simulink model "ClosedLoopControl"  (R2016b)
settings: Solver=FixedStepDiscrete  StartTime=0.0  StopTime=Inf  FixedStep=sCoreParams.core.stepPeriod  RelTol=1e-3  EnableMultiTasking=on
undefined symbols (not defined in the file): fdesignblkfcn, gcbh, High, sCoreParams, sCoreParams_decoders_chanceDetector_randStimEventsPerSec, sCoreParams_decoders_txDetector_channel1, sCoreParams_decoders_txDetector_channel2, sCoreParams_decoders_txDetector_detectChannelInds, sCoreParams_decoders_txDetector_nChannels, sCoreParams_Features_Baseline_initialThresholdValue, sCoreParams_Features_Baseline_weightPreviousThreshold, sCoreParams_Features_Data_SmoothWindowsDurationSamples, sCoreParams_stimulator_stimAfterDelaySteps
libraries: dsparch4 x20, dspstat3 x19, dspspect3 x6, dspfdesign x2, dspindex x2, dspswit3 x1
(part 3 of 6)

== system ClosedLoopControl/FilterBanks/Variant FILTER 1000/4-8Hz Theta FIR ==
  EEGData : Inport
  Generated Filter Block : DiscreteFir  Tag=BlockMethodSubSystem  Coefficients=[-4.0965914206968854e-05 -3.1562576663732106e-05 -2.1885911724999518e-05 -1.1939596349254351e-05 -1.7275529186717732e-06 8.7460521918561927e-06 1.947681025149899e-05 3.0460072015961004e-05 4.1690949775364282e-05 5.316431960704088e-05 6.4874823832640496e-05 7.6816873678724166e-05 8.8984652139878232e-05 0.00010137211704322235 0.00011397300431296607 0.00012678083143356132 0.00013978890110980167 0.00015299030512201677 0.0001663779283744122 0.00017994445313437968 0.00019368236346045136 0.00020758394981644162 0.00022164131386907284 0.00023584637346632409 0.00025019086779349122 0.00026466636270383186 0.00027926425622051192 0.00029397578420637229 0.0003087920261979428 0.00032370391139992542 0.00033870222483622773 0.00035377761365352274 0.00036892059357309124 0.00038412155548662883 0.00039937077219152613 0.00041465840526098188 0.00042997451204421873 0.00044530905279189289 0.00046065189790167919 0.00047599283527891651 0.00049132157780700891 0.00050662777092225068 0.00052190100028754523 0.00053713079955942423 0.0005523066582426813 0.00056741802962677009 0.00058245433879808891 0.000597404990722145 0.00061225937838948802 0.00062700689101926807 0.00064163692231413751 0.0006561388787601712 0.00067050218796541777 0.00068471630703058827 0.00069877073094537284 0.00071265500100379619 0.00072635871323196185 0.00073987152682152089 0.00075318317256212598 0.00076628346126611058 0.00077916229217862127 0.00079180966136635381 0.00080421567007808498 0.00081637053307013834 0.00082826458688991199 0.00083988829811062636 0.0008512322715104072 0.00086228725818885592 0.00087304416361427394 0.00088349405559469028 0.00089362817216592349 0.00090343792938986952 0.00091291492905630825 0.00092205096628152127 0.00093083803699705442 0.0009392683453220477 0.00094733431081258041 0.00095502857558154447 0.00096234401128264535 0.00096927372595218225 0.00097581107070235091 0.0009819496462598993 0.00098768330934403915 0.00099300617887762544 0.00099791264202572761 0.0010023973600557757 0.0010064552740136482 0.0010100816102101011 0.0010132718855121318 0.001016021912433947 0.0010183278040223579 0.0010201859785315629 0.001021593163882393 0.0010225464019012794 0.0010230430523343159 0.0010230807966319598 0.0010226576415000763 0.0010217719222131735 0.0010204223056858744 0.0010186077932988016 0.0010163277234752684 0.0010135817740053027 0.001010369964113756 0.0010066926562693997 0.0010025505577321177 0.00099794472183549455 0.00099287654900228565 0.00098734778749046018 0.00098136053386771059 0.00097491723321251631 0.00096802067904005952 0.00096067401295151704 0.00095288072400541532 0.0009446446478100181 0.0009359699653358561 0.00092686120144778344 0.0009173232231561401 0.00090736123758679863 0.00089698078967015025 0.00088618775954923501 0.00087498835970750667 0.00086338913181691805 0.00085139694330722165 0.00083901898365764142 0.00082626276041227885 0.00081313609492081231 0.00079964711780634835 0.00078580426416241132 0.00077161626848136554 0.0007570921593167498 0.00074224125368220961 0.00072707315118998063 0.00071159772793206099 0.00069582513010743195 0.00067976576739893664 0.00066343030610358899 0.00064682966202034113 0.00062997499309955815 0.0006128776918585834 0.00059554937756810765 0.00057800188821412754 0.00056024727224058429 0.00054229778007792984 0.00052416585546304225 0.00050586412655614986 0.00048740539686060552 0.00046880263595147945 0.00045006897001921846 0.00043121767223470618 0.00041226215294230351 0.00039321594968756213 0.00037409271708650435 0.00035490621654351472 0.0003356703058250473 0.00031639892849649162 0.00029710610322969557 0.00027780591298878944 0.00025851249410209314 0.0002392400252279985 0.00022000271622286136 0.00020081479691906072 0.00018169050582149475 0.00016264407873087066 0.00014368973730227231 0.00012484167754757907 0.00010611405829039998 8.7520989582255267e-05 6.9076521088845522e-05 5.0794630455274516e-05 3.268921165922444e-05 1.4774063361054236e-05 -2.937122740077089e-06 -2.0430773534982893e-05 -3.7693446108933282e-05 -5.4711839312708335e-05 ...(+22999 chars)]  InputProcessing=Columns as channels (frame based)
  filteredData : Outport
  wires:
  EEGData/1 -> Generated Filter Block/1
  Generated Filter Block/1 -> filteredData/1

== system ClosedLoopControl/FilterBanks/Variant FILTER 1000/4-8Hz Theta IIR ==
  EEGData : Inport
  Generated Filter Block : dsparch4/Biquad Filter  Tag=BlockMethodSubSystem  IIRFiltStruct=Direct form II  CoeffSource=Specify via dialog  BiQuadCoeffs=[0.06931048107077438 0 -0.06931048107077438 1 -1.9802222626264796 0.98069219275950414;0.018212718480246574 0 -0.018212718480246574 1 -1.974229549932226 0.97738422717098938;0.023158348233385473 0 -0.023158348233385473 1 -1.9641498959199661 0.96500779271339332;0.0024959904089144444 0 -0.0024959904089144444 1 -1.9561756271771134 0.95744921192041055;0.0038077695663208747 0 -0.0038077695663208747 1 -1.997161027977103 0.9974982403948508;0.014974735737014893 0 -0.014974735737014893 1 -1.9920313655652335 0.99238598997351135;0.067760808502200814 0 -0.067760808502200814 1 -1.9727869770434667 0.9733937566537022;0.057203187978703156 0 -0.057203187978703156 1 -1.9624464044097747 0.96525472973103199;0.04408340167774278 0 -0.04408340167774278 1 -1.9548134348661885 0.95715627089409527;0.057491867954990714 0 -0.057491867954990714 1 -1.9525307286276412 0.95433606793971626;0.0088260244022239226 0 -0.0088260244022239226 1 -1.9887766913282909 0.99212744222685822;2 0 -2 1 -1.9865011906165977 0.98689604525630514]  a0Flag=Warning  IC=0  ICnum=0  ICden=0  InputProcessing=Columns as channels (frame based)  denAccumFracLength=30  denProdOutputFracLength=30  secondMemoryFracLength=15  roundingMode=Floor  overflowMode=off  ScaleValues=[0.00037611451030394085;1;1;1;1;1;1;1;1;1;1;1;12.523892689936686]  optimizeScaleValues=off  ScaleValueMode=Specify via input port (g)  scaleValueFracLength=14  FilterSource=Specify via dialog  FilterObject=BQF
  filteredData : Outport
  wires:
  EEGData/1 -> Generated Filter Block/1
  Generated Filter Block/1 -> filteredData/1

== system ClosedLoopControl/FilterBanks/Variant FILTER 1000/65-110Hz HighGamma FIR ==
  EEGData : Inport
  Generated Filter Block : DiscreteFir  Tag=BlockMethodSubSystem  Coefficients=[0.013804330140111717 -0.0032030301327593746 -0.0026076510316669732 -0.0019065599324483403 -0.0010950973516722739 -0.00016216284695244599 0.00086566972400229725 0.0019516885555648496 0.0030106913379105565 0.0039390669121143725 0.0046071460998753817 0.0048943907316536354 0.0046884459511977224 0.0039269229728160996 0.0025931297718577782 0.00075000967683423552 -0.0014812603255484518 -0.0039070830585515659 -0.0062985241582419948 -0.0083973498946592028 -0.0099678263784681084 -0.010809035903715401 -0.010803230740337099 -0.0099149025044472407 -0.0082222253166924462 -0.0058958474615859622 -0.0031966951596653086 -0.00042921572872034144 0.0020843075499259859 0.0040591524840028152 0.005272016533938776 0.0056235264011517839 0.0051356663591639361 0.0039469466526657771 0.0023736337698522614 0.00069406556447416045 -0.00062224964462739992 -0.0012265818590162169 -0.00086373706682174275 0.00064926343879799649 0.0032891772017854025 0.0068616007904351807 0.010959888764209976 0.015047965951643011 0.018483860601451012 0.020629088707457537 0.020895258620364673 0.018864941232038121 0.014327792052099074 0.0073683568396857536 -0.0016488647216768106 -0.012058123582057797 -0.022974047895930626 -0.033340495226029006 -0.042069205650392676 -0.048123624580120594 -0.050670829782113042 -0.04915218268598933 -0.043397073906481516 -0.033631108507841165 -0.020501148353700021 -0.0049965672361083416 0.011603807282296149 0.02788293342498982 0.042383528564973294 0.053814263792701968 0.061127840120098795 0.06363510173931633 0.061127840120098795 0.053814263792701968 0.042383528564973294 0.02788293342498982 0.011603807282296149 -0.0049965672361083416 -0.020501148353700021 -0.033631108507841165 -0.043397073906481516 -0.04915218268598933 -0.050670829782113042 -0.048123624580120594 -0.042069205650392676 -0.033340495226029006 -0.022974047895930626 -0.012058123582057797 -0.0016488647216768106 0.0073683568396857536 0.014327792052099074 0.018864941232038121 0.020895258620364673 0.020629088707457537 0.018483860601451012 0.015047965951643011 0.010959888764209976 0.0068616007904351807 0.0032891772017854025 0.00064926343879799649 -0.00086373706682174275 -0.0012265818590162169 -0.00062224964462739992 0.00069406556447416045 0.0023736337698522614 0.0039469466526657771 0.0051356663591639361 0.0056235264011517839 0.005272016533938776 0.0040591524840028152 0.0020843075499259859 -0.00042921572872034144 -0.0031966951596653086 -0.0058958474615859622 -0.0082222253166924462 -0.0099149025044472407 -0.010803230740337099 -0.010809035903715401 -0.0099678263784681084 -0.0083973498946592028 -0.0062985241582419948 -0.0039070830585515659 -0.0014812603255484518 0.00075000967683423552 0.0025931297718577782 0.0039269229728160996 0.0046884459511977224 0.0048943907316536354 0.0046071460998753817 0.0039390669121143725 0.0030106913379105565 0.0019516885555648496 0.00086566972400229725 -0.00016216284695244599 -0.0010950973516722739 -0.0019065599324483403 -0.0026076510316669732 -0.0032030301327593746 0.013804330140111717]  InputProcessing=Columns as channels (frame based)
  filteredData : Outport
  wires:
  EEGData/1 -> Generated Filter Block/1
  Generated Filter Block/1 -> filteredData/1

== system ClosedLoopControl/FilterBanks/Variant FILTER 1000/65-110Hz HighGamma IIR ==
  EEGData : Inport
  Generated Filter Block : dsparch4/Biquad Filter  Tag=BlockMethodSubSystem  IIRFiltStruct=Direct form II  CoeffSource=Specify via dialog  BiQuadCoeffs=[0.068135075292954525 0 -0.068135075292954525 1 -1.7248750360257281 0.90187102511020312;0.14832830488548138 0 -0.14832830488548138 1 -1.6834117803685955 0.86637329099306459;0.21032334743416023 0 -0.21032334743416023 1 -1.5199665196913907 0.76281126114730169;0.24002790188276571 0 -0.24002790188276571 1 -1.4386332473664822 0.76228280789590785;0.098329082421743721 0 -0.098329082421743721 1 -1.430740080325084 0.81486233962044397;0.017120606387656199 0 -0.017120606387656199 1 -1.5993559620394144 0.80472299209173781;0.34252166100538306 0 -0.34252166100538306 1 -1.8047004225280108 0.97943124566931283;0.30513864191887496 0 -0.30513864191887496 1 -1.5087272028926828 0.96803465980821457;0.089298096792288673 0 -0.089298096792288673 1 -1.4443882700966519 0.8570440761411624;0.17963067322639797 0 -0.17963067322639797 1 -1.6413615575457359 0.83370854118735804;0.20371135066215332 0 -0.20371135066215332 1 -1.4858612806505964 0.75293305209773154;0.19033988234903718 0 -0.19033988234903718 1 -1.4581042693456889 0.75240497690189601;0.11355284823690669 0 -0.11355284823690669 1 -1.4290957907835335 0.78310330426719232;0.046342840146937798 0 -0.046342840146937798 1 -1.5584074492012501 0.78060128626386927;0.31365056915550737 0 -0.31365056915550737 1 -1.7653830457658011 0.93966121683222037;1.1749399341551727 0 -1.1749399341551727 1 -1.4704231296619215 0.90862777392305505]  a0Flag=Warning  IC=0  ICnum=0  ICden=0  InputProcessing=Columns as channels (frame based)  denAccumFracLength=30  denProdOutputFracLength=30  secondMemoryFracLength=15  roundingMode=Floor  overflowMode=off  ScaleValues=[0.041082197949265611;1;1;1;1;1;1;1;1;1;1;1;1;1;1;1;1]  optimizeScaleValues=off  ScaleValueMode=Specify via input port (g)  scaleValueFracLength=14  FilterSource=Specify via dialog  FilterObject=BQF
  filteredData : Outport
  wires:
  EEGData/1 -> Generated Filter Block/1
  Generated Filter Block/1 -> filteredData/1

== system ClosedLoopControl/FilterBanks/Variant FILTER 1000/65-200Hz HighGammaRipple FIR ==
  EEGData : Inport
  Generated Filter Block : DiscreteFir  Tag=BlockMethodSubSystem  Coefficients=[0.043674950645707943 -0.010510801076776438 -0.0092198604406533054 -0.0078072197440863019 -0.0061576291109547441 -0.0043314949479796505 -0.0026149837714866844 -0.0014281197315007387 -0.0011887830977032846 -0.0020631394359844836 -0.0038906609829976006 -0.006134979543899413 -0.0080743521554436769 -0.0090186910392010006 -0.0085928718984132329 -0.0068824719973744029 -0.0044344002598706734 -0.0020632098371482117 -0.00054620058864337216 -0.00031706926836648172 -0.0012806039208504247 -0.0028303540771732584 -0.0040768356042938676 -0.004193132697654047 -0.0027660676413756961 1.9003693936618729e-05 0.0034067519279456487 0.0063472526354222602 0.0078958974614977504 0.0075793823939889725 0.0056281036442865778 0.0028514070097576216 0.00042987516134896416 -0.00071303834093239911 1.1697363323633972e-05 0.0020369008242335485 0.0045707172575817877 0.0063400232285504843 0.006152335767163339 0.003695198751154251 -0.00054923784249524951 -0.0052930021300986009 -0.009082894815013105 -0.010679189468049901 -0.009713948692912408 -0.0067468353855187129 -0.0031802128714443988 -0.00063228620545409213 -0.00035139072256231481 -0.0026086409852362456 -0.0065830274486462651 -0.010571501918713583 -0.012689614383126465 -0.011577477565379819 -0.0070576745373317736 -0.00022999532853976319 0.0068154951113979841 0.011843234875324286 0.013289460151243533 0.011001391875699177 0.0063095176650106582 0.0016313362199767314 -0.00052119400123590027 0.0014569178651438908 0.0074726777669980133 0.015628713969671838 0.022826703629726497 0.025893486581749524 0.022907578453487763 0.014019972540609493 0.0016645482174998925 -0.010167457554019462 -0.017562158381230882 -0.0180477323755667 -0.01194498020464765 -0.0024264873025872094 0.0052207045747070255 0.0056493327084122186 -0.0045373885153166225 -0.025015012812241458 -0.051246002878708945 -0.075349015080128312 -0.088355355358379697 -0.083035398155685114 -0.056553784398185536 -0.011862247095400281 0.042515847778265718 0.094576601537287724 0.13197925194672577 0.14558091380700244 0.13197925194672577 0.094576601537287724 0.042515847778265718 -0.011862247095400281 -0.056553784398185536 -0.083035398155685114 -0.088355355358379697 -0.075349015080128312 -0.051246002878708945 -0.025015012812241458 -0.0045373885153166225 0.0056493327084122186 0.0052207045747070255 -0.0024264873025872094 -0.01194498020464765 -0.0180477323755667 -0.017562158381230882 -0.010167457554019462 0.0016645482174998925 0.014019972540609493 0.022907578453487763 0.025893486581749524 0.022826703629726497 0.015628713969671838 0.0074726777669980133 0.0014569178651438908 -0.00052119400123590027 0.0016313362199767314 0.0063095176650106582 0.011001391875699177 0.013289460151243533 0.011843234875324286 0.0068154951113979841 -0.00022999532853976319 -0.0070576745373317736 -0.011577477565379819 -0.012689614383126465 -0.010571501918713583 -0.0065830274486462651 -0.0026086409852362456 -0.00035139072256231481 -0.00063228620545409213 -0.0031802128714443988 -0.0067468353855187129 -0.009713948692912408 -0.010679189468049901 -0.009082894815013105 -0.0052930021300986009 -0.00054923784249524951 0.003695198751154251 0.006152335767163339 0.0063400232285504843 0.0045707172575817877 0.0020369008242335485 1.1697363323633972e-05 -0.00071303834093239911 0.00042987516134896416 0.0028514070097576216 0.0056281036442865778 0.0075793823939889725 0.0078958974614977504 0.0063472526354222602 0.0034067519279456487 1.9003693936618729e-05 -0.0027660676413756961 -0.004193132697654047 -0.0040768356042938676 -0.0028303540771732584 -0.0012806039208504247 -0.00031706926836648172 -0.00054620058864337216 -0.0020632098371482117 -0.0044344002598706734 -0.0068824719973744029 -0.0085928718984132329 -0.0090186910392010006 -0.0080743521554436769 -0.006134979543899413 -0.0038906609829976006 -0.0020631394359844836 -0.0011887830977032846 -0.0014281197315007387 -0.0026149837714866844 -0.0043314949479796505 -0.0061576291109547441 -0.0078072197440863019 -0.0092198604406533054 -0.010510801076776438 0.043674950645707943]  InputProcessing=Columns as channels (frame based)
  filteredData : Outport
  wires:
  EEGData/1 -> Generated Filter Block/1
  Generated Filter Block/1 -> filteredData/1

== system ClosedLoopControl/FilterBanks/Variant FILTER 1000/65-200Hz HighGammaRipple IIR ==
  EEGData : Inport
  Generated Filter Block : dsparch4/Biquad Filter  Tag=BlockMethodSubSystem  IIRFiltStruct=Direct form II  CoeffSource=Specify via dialog  BiQuadCoeffs=[0.53247966268348346 0 -0.53247966268348346 1 -0.52704151476078853 0.73570357892148941;0.35902600784170141 0 -0.35902600784170141 1 -1.5290645007219816 0.71654477045619724;0.38930274708430884 0 -0.38930274708430884 1 -1.0674429840511706 0.40759732672655757;0.28894721065879136 0 -0.28894721065879136 1 -0.68462766684650866 0.36375649736693272;0.37967452704956917 0 -0.37967452704956917 1 -1.3302818606200466 0.56022088202635434;0.11007109362133076 0 -0.11007109362133076 1 -0.55801925843952827 0.49572700074922765;0.38533235757507273 0 -0.38533235757507273 1 -1.7773213023068468 0.9562473271848021;0.52082665364290004 0 -0.52082665364290004 1 -0.55181079637462238 0.90253323762634019;0.19994668477824018 0 -0.19994668477824018 1 -1.4355646668071909 0.63899712759644189;0.41392191533089728 0 -0.41392191533089728 1 -0.53033830788206182 0.60149793516900418;0.38066692212958297 0 -0.38066692212958297 1 -0.91955821846029517 0.35630842395845075;0.46576541117451042 0 -0.46576541117451042 1 -0.78790513173646048 0.34173908145142229;0.3020569205846822 0 -0.3020569205846822 1 -1.2082108913787444 0.48093385694549734;0.57198921484629695 0 -0.57198921484629695 1 -0.60901125444153781 0.41631824434388354;0.25422736500537629 0 -0.25422736500537629 1 -1.6969384082346077 0.87321629135880463;1.1213529185216204 0 -1.1213529185216204 1 -1.6150827711889018 0.79402829840242117]  a0Flag=Warning  IC=0  ICnum=0  ICden=0  InputProcessing=Columns as channels (frame based)  denAccumFracLength=30  denProdOutputFracLength=30  secondMemoryFracLength=15  roundingMode=Floor  overflowMode=off  ScaleValues=[0.25151386008232818;1;1;1;1;1;1;1;1;1;1;1;1;1;1;1;1]  optimizeScaleValues=off  ScaleValueMode=Specify via input port (g)  scaleValueFracLength=14  FilterSource=Specify via dialog  FilterObject=BQF
  filteredData : Outport
  wires:
  EEGData/1 -> Generated Filter Block/1
  Generated Filter Block/1 -> filteredData/1
